simulink model "akm_simulink"  (R2021b)
settings: Solver=ode45  StartTime=0.0  StopTime=10.0  RelTol=1e-3
settings Model: Creator=86188  LastModifiedBy=ASUS
settings SolverCC: AlgebraicLoopSolver=TrustRegion
settings DataIOCC: LimitDataPoints=on  SaveFormat=Array  ReturnWorkspaceOutputs=off
settings OptimizationCC: BlockReduction=off  BooleanDataType=off  LifeSpan=inf
settings DebuggingCC: SaveWithParameterizedLinksMsg=none  UnderspecifiedInitializationDetection=Classic  MergeDetectMultiDrivingBlocksExec=none  SignalResolutionControl=TryResolveAllWithWarning  SFUnexpectedBacktrackingDiag=warning  SFNoUnconditionalDefaultTransitionDiag=warning  SFExecutionAtInitializationDiag=none  SFMachineParentedDataDiag=warning  ArithmeticOperatorsInVariantConditions=warning
settings HardwareCC: ProdBitPerPointer=32  ProdBitPerSizeT=32  ProdBitPerPtrDiffT=32  ProdLargestAtomicFloat=None  ProdIntDivRoundTo=Undefined  ProdEndianess=Unspecified  ProdWordSize=32  ProdHWDeviceType=32-bit Generic  TargetUnknown=on
settings ModelReferenceCC: PropagateSignalLabelsOutOfModel=off
settings SFSimCC: SimUseLocalCustomCode=off  CustomCodeUndefinedFunction=UseInterfaceOnly
settings RTWCC: RTWUseLocalCustomCode=off
settings CodeAppCC: StateflowObjectComments=on
settings GRTTargetCC: TargetLangStandard=C89/C90 (ANSI)
settings ConfigComp: CovMetricSettings=dw  CovSaveCumulativeToWorkspaceVar=on  CovSaveSingleToWorkspaceVar=on  CovExternalEMLEnable=off  CovSFcnEnable=off

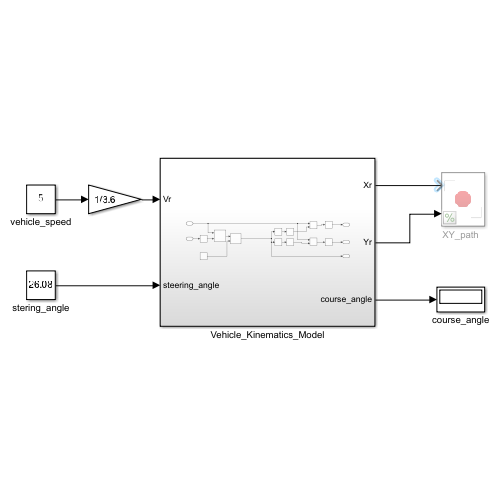
[thumbnail: Simulink's stored preview of the top-level diagram]
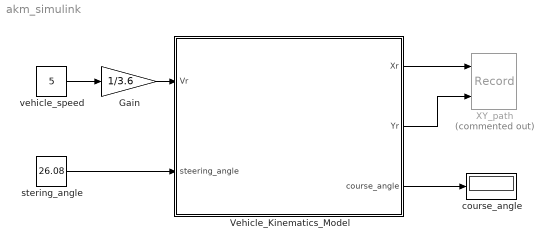
== system akm_simulink ==
  Gain : Gain  Gain=1/3.6
  Vehicle_Kinematics_Model : Subsystem
  "XY_path  " : Record  Commented=on  FileSettingsInternal="{\"entries\":[{\"content\":{\"excelSettings\":{\"content\":{},\"type\":\"Streamout.ExcelSettings\"}},\"type\":\"Streamout.FileSettingStorage\",\"uuid\":\"7addfd98-46f2-4b72-a359-b2e0c588f249\"}],\"packageUris\":[\"http://schema.mathworks.com/mf0/streamout_blocks/R2020a\"],\"version\":\"1.0\"}"  Layout=[1 1]  SignalsInternal="{\"entries\":[{\"content\":{\"signals\":[{\"content\":{\"blockPath\":[\"vehicle_kinematics_model_simulink/XY_path  \"],\"channel\":[],\"dimensions\":[1],\"domain\":\"vehicle_kinematics_model_simulink/XY_path  \",\"lineColor\":\"#a2142f\",\"plots\":[1],\"port\":1,\"sid\":[],\"signalID\":25,\"signalName\":\"XY Graph:1\"},\"type\":\"RecordBlkView.Signal\",\"uuid\":\"aea1348b-08f8-4aad-b363-d4c46aa4d93b\"},{\"content\":{\"blockPath\":[\"vehicle_kinematics_model_simulink/XY_path  \"],\"channel\":[],\"dimensions\":[1],\"domain\":\"vehicle_kinematics_model_simulink/XY_path  \",\"lineColor\":\"#139fff\",\"plots\":[1],\"port\":2,\"sid\":[],\"signalID\":28,\"signalName\":\"XY Graph:2\"},\"type\":\"RecordBlkView.Signal\",\"uuid\":\"a975d67e-8dd6-489c-87d0-dd0b00579815\"}]},\"type\":\"RecordBlkView.InputSignals\",\"uuid\":\"86e3c1e8-de57-43d6-8970-4e9e7abf98df\"}],\"packageUris\":[\"http://schema.mathworks.com/mf0/streamout_blocks/R2020a\"],\"version\":\"1.0\"}"  VisualizationBindings="{\"xyplotplugin\":{\"info\":[{\"series\":[{\"bindingParametersList\":[{\"parameter\":\"X-Axis\",\"signalID\":25,\"signalName\":\"XY Graph:1\"},{\"parameter\":\"Y-Axis\",\"signalID\":28,\"signalName\":\"XY Graph:2\"}],\"seriesID\":38578}],\"subplotID\":1}]}}"  CompatibilityTag=XY  st=-1
  course_angle : Display
  stering_angle : Constant  Value=26.08
  vehicle_speed : Constant  Value=5
  wires:
  Gain/1 -> Vehicle_Kinematics_Model/1(Vr)
  stering_angle/1 -> Vehicle_Kinematics_Model/2(steering_angle)
  vehicle_speed/1 -> Gain/1
  Vehicle_Kinematics_Model/2(Yr) -> "XY_path  "/2
  Vehicle_Kinematics_Model/1(Xr) -> "XY_path  "/1
  Vehicle_Kinematics_Model/3(course_angle) -> course_angle/1

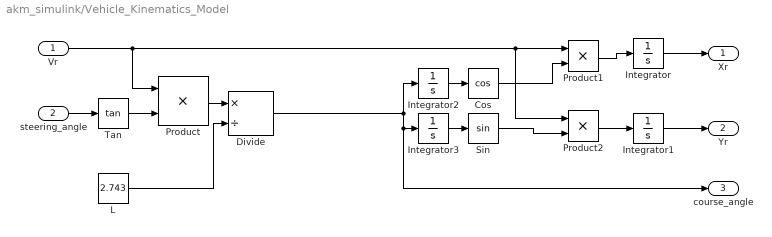
== system akm_simulink/Vehicle_Kinematics_Model ==
  Vr : Inport
  steering_angle : Inport  Port=2
  Cos : Trigonometry  Operator=cos
  Divide : Product  Inputs=*/
  Integrator{,1..3} (4 alike) : Integrator
  L : Constant  Value=2.743
  Product : Product
  Product1 : Product
  Product2 : Product
  Sin : Trigonometry
  Tan : Trigonometry  Operator=tan
  Xr : Outport
  Yr : Outport  Port=2
  course_angle : Outport  Port=3
  wires:
  Product2/1 -> Integrator1/1
  Product1/1 -> Integrator/1
  Sin/1 -> Product2/2
  L/1 -> Divide/2
  Integrator1/1 -> Yr/1
  Tan/1 -> Product/2
  Integrator/1 -> Xr/1
  Product/1 -> Divide/1
  steering_angle/1 -> Tan/1
  Divide/1 -> Integrator2/1, course_angle/1, Integrator3/1
  Cos/1 -> Product1/2
  Vr/1 -> Product/1, Product1/1, Product2/1
  Integrator2/1 -> Cos/1
  Integrator3/1 -> Sin/1
